simulink model "SerieRuidoEntrada2"  (Simulink 7.5)
settings: Solver=ode3  StartTime=Intime  StopTime=Sttime  FixedStep=stime  RelTol=1e-3
values from neighbouring files (symbols this model uses):
  FTf = 1/mag*FTfp    [Filtros.m]    (also in RuidoFiltroN.m)
  FTf2 = 1/mag2*FTfp2    [Filtros.m]    (also in RuidoFiltroN.m)
  FTf3 = 1/mag3*FTfp3    [Filtros.m]
  Intime = 0    [Filtros.m]    (also in RuidoFiltroN.m)
  Sttime = 40    [Filtros.m]    (also in RuidoFiltroN.m = 20)
  t2 = 15    [Filtros.m]
  t3 = 30    [Filtros.m]
libraries: simulink x1
settings Model: Creator=Ferdinando  LastModifiedBy=Ferdinando

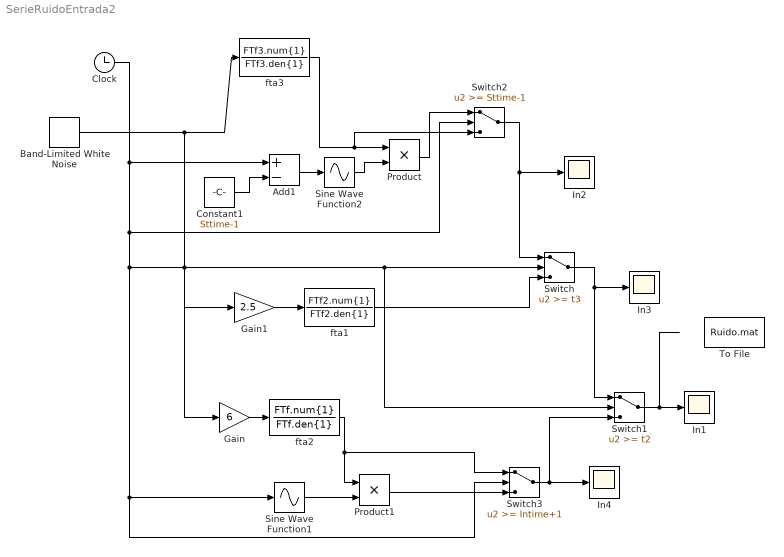
== system SerieRuidoEntrada2 ==
  Add1 : Sum  Inputs=+-  OutDataType=sfix(16)  OutScaling=2^-10
  Band-Limited White Noise : simulink/Sources/Band-Limited White Noise  SystemSampleTime=-1  Cov=[3.163*10^-5]  Ts=10^-3  seed=[23341]
  Clock : Clock
      settings: Decimation=10
  Constant1 : Constant  Value=Sttime-1  OutDataType=sfix(16)  OutScaling=2^0
  Gain : Gain  Gain=6  ParameterDataType=fixdt(1, 16)  ParameterScaling=2^0  OutDataType=fixdt(1, 16)  OutScaling=2^0
  Gain1 : Gain  Gain=2.5  ParameterDataType=fixdt(1, 16)  ParameterScaling=2^0  OutDataType=fixdt(1, 16)  OutScaling=2^0
  In{1..4} (4 alike) : Scope
      In1 settings: SaveName=Rand3and
      In2 settings: SaveName=Rand3and1
      In3 settings: SaveName=Rand3and2
      In4 settings: SaveName=Rand3and3
  Product : Product  OutDataType=sfix(16)  OutScaling=2^0  RndMeth=Zero
  Product1 : Product  OutDataType=sfix(16)  OutScaling=2^0  RndMeth=Zero
  Sine Wave Function1 : Sin  TimeSource=Use external signal  Amplitude=0.5  Bias=0.5  Frequency=pi  Phase=-pi/2  Samples=10  SampleTime=0  Offset=0
  Sine Wave Function2 : Sin  TimeSource=Use external signal  Amplitude=0.5  Bias=0.5  Frequency=pi  Phase=pi/2  Samples=10  SampleTime=0  Offset=0
  Switch : Switch  Threshold=t3  OutDataType=fixdt(1, 16)  OutScaling=2^0
  Switch1 : Switch  Threshold=t2  OutDataType=fixdt(1, 16)  OutScaling=2^0
  Switch2 : Switch  Threshold=Sttime-1  OutDataType=fixdt(1, 16)  OutScaling=2^0
  Switch3 : Switch  Threshold=Intime+1  OutDataType=fixdt(1, 16)  OutScaling=2^0
  To File : ToFile  Filename=Ruido.mat  MatrixName=Ruido
  fta1 : TransferFcn  Numerator=FTf2.num{1}  Denominator=FTf2.den{1}
  fta2 : TransferFcn  Numerator=FTf.num{1}  Denominator=FTf.den{1}
  fta3 : TransferFcn  Numerator=FTf3.num{1}  Denominator=FTf3.den{1}
  wires:
  Band-Limited White Noise/1 -> Gain1/1, Gain/1, fta3/1
  Clock/1 -> Add1/1, Switch/2, Switch1/2, Switch3/2, Sine Wave Function1/1, Switch2/2
  fta1/1 -> Switch/3
  Switch/1 -> Switch1/1, In3/1
  Switch1/1 -> In1/1
  Gain1/1 -> fta1/1
  Gain/1 -> fta2/1
  Sine Wave Function2/1 -> Product/2
  fta3/1 -> Product/1, Switch2/3
  Product/1 -> Switch2/1
  Switch2/1 -> Switch/1, In2/1
  Switch3/1 -> Switch1/3, In4/1
  Sine Wave Function1/1 -> Product1/2
  fta2/1 -> Product1/1, Switch3/1
  Add1/1 -> Sine Wave Function2/1
  Constant1/1 -> Add1/2
  Product1/1 -> Switch3/3
